simulink model "pratica2_1_b"  (R2021a)
settings: Solver=VariableStepAuto  StartTime=0.0  StopTime=10.0  RelTol=1e-3
libraries: fl_lib x11, ee_lib x7, nesl_utility x2
settings Model: Creator=ribeiro  LastModifiedBy=ribeiro

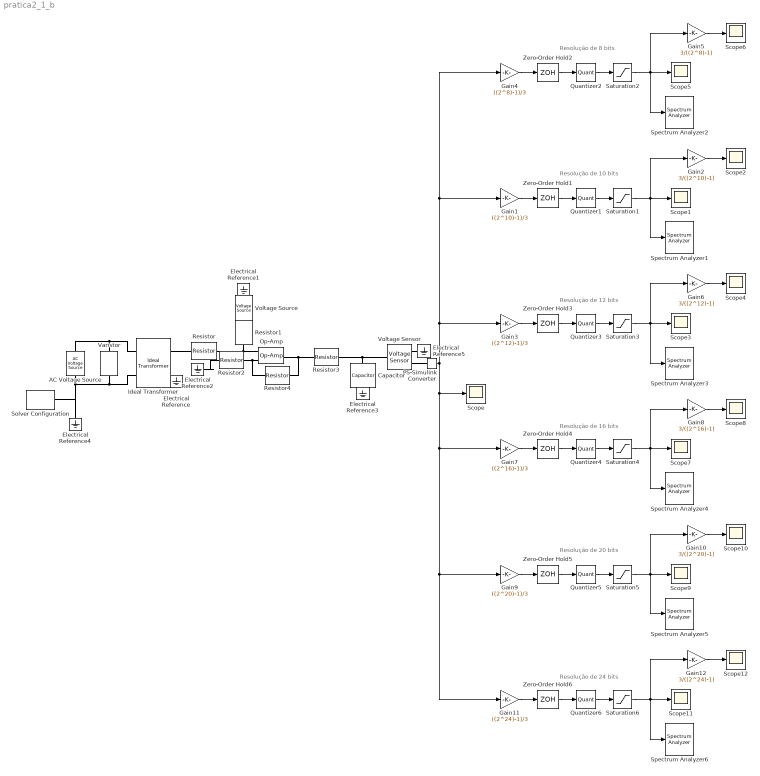
== system pratica2_1_b ==
  note: Resolução de 8 bits
  note: Resolução de 10 bits
  note: Resolução de 12 bits
  note: Resolução de 16 bits
  note: Resolução de 20 bits
  note: Resolução de 24 bits
  AC Voltage Source : fl_lib/Electrical/Electrical Sources/AC Voltage Source  amp=180 V  shift=0 deg  frequency=60 Hz  omega=0 rad/s
  Capacitor : fl_lib/Electrical/Electrical Elements/Capacitor  c=3.2 uF  r=1e-6 Ohm  g=0 1/Ohm  i_specify=off  i_priority=None  i=0 A  i_nominal_specify=off  i_nominal_unit=A  i_nominal_value=1  v_specify=off  v_priority=None  v=0 V  v_nominal_specify=off  v_nominal_unit=V  v_nominal_value=1  vc_specify=off  vc_priority=High  vc=0 V  vc_nominal_specify=off  vc_nominal_unit=V  vc_nominal_value=1
  Electrical Reference{,1..5} (6 alike) : fl_lib/Electrical/Electrical Elements/Electrical Reference
  Gain1 : Gain  Gain=((2^10)-1)/3
  Gain10 : Gain  Gain=3/((2^20)-1)
  Gain11 : Gain  Gain=((2^24)-1)/3
  Gain12 : Gain  Gain=3/((2^24)-1)
  Gain2 : Gain  Gain=3/((2^10)-1)
  Gain3 : Gain  Gain=((2^12)-1)/3
  Gain4 : Gain  Gain=((2^8)-1)/3
  Gain5 : Gain  Gain=3/((2^8)-1)
  Gain6 : Gain  Gain=3/((2^12)-1)
  Gain7 : Gain  Gain=((2^16)-1)/3
  Gain8 : Gain  Gain=3/((2^16)-1)
  Gain9 : Gain  Gain=((2^20)-1)/3
  Ideal Transformer : fl_lib/Electrical/Electrical Elements/Ideal Transformer  n=120/1  i1_specify=off  i1_priority=None  i1=0 A  i1_nominal_specify=off  i1_nominal_unit=A  i1_nominal_value=1  v1_specify=off  v1_priority=None  v1=0 V  v1_nominal_specify=off  v1_nominal_unit=V  v1_nominal_value=1  i2_specify=off  i2_priority=None  i2=0 A  i2_nominal_specify=off  i2_nominal_unit=A  i2_nominal_value=1  v2_specify=off  v2_priority=None  v2=0 V  v2_nominal_specify=off  v2_nominal_unit=V  v2_nominal_value=1
      settings: SourceProductBaseCode=SS
  Op-Amp : fl_lib/Electrical/Electrical Elements/Op-Amp  outI_specify=off  outI_priority=None  outI=0 A  outI_nominal_specify=off  outI_nominal_unit=A  outI_nominal_value=1
  PS-Simulink Converter : nesl_utility/PS-Simulink Converter  PhysicalDomain=network_engine_domain  SubClassName=ps_output  LeftPortType=input  RightPortType=output  PseudoPeriodic=off  Frequencies=[]  Unit=inherit  AffineConversion=off
      settings: SourceProductBaseCode=PW,SS
  Quantizer1 : Quantizer  QuantizationInterval=1/((2^10)-1)
  Quantizer2 : Quantizer  QuantizationInterval=1/((2^8)-1)
  Quantizer3 : Quantizer  QuantizationInterval=1/((2^12)-1)
  Quantizer4 : Quantizer  QuantizationInterval=1/((2^16)-1)
  Quantizer5 : Quantizer  QuantizationInterval=1/((2^20)-1)
  Quantizer6 : Quantizer  QuantizationInterval=1/((2^24)-1)
  Resistor : ee_lib/Passive/Resistor  R=10 kOhm  R_tol=5  enable_R_tol=0  tol_distribution=1  nSigma=4  enable_operating_limits=0  operating_limit_action=2  max_working_voltage=100 V  power_rating=1 W  enable_faults=0  fault_action=1  R_faulted=inf Ohm  enable_temporal_fault=0  t_fault=1 s  enable_behavioral_fault=0  max_permissible_current=1 A  t_fail_on_current=1 s  noise_mode=0  sample_time=1e-3 s  repeatability=1  auto_seed=3546856910  user_seed=0  Tdevice=25 degC  alpha=3.93e-3 1/K  Tmeas=25 degC  thermal_mass=100 J/K  power_derating_T1=70 degC  power_derating_T2=155 degC  operating_temperature_range_vec=[-50, 150] degC  temperature_specify=off  temperature_priority=High  temperature=298.15 K  temperature_nominal_specify=off  temperature_nominal_unit=K  temperature_nominal_value=1
  Resistor1 : ee_lib/Passive/Resistor  R=10 kOhm  R_tol=5  enable_R_tol=0  tol_distribution=1  nSigma=4  enable_operating_limits=0  operating_limit_action=2  max_working_voltage=100 V  power_rating=1 W  enable_faults=0  fault_action=1  R_faulted=inf Ohm  enable_temporal_fault=0  t_fault=1 s  enable_behavioral_fault=0  max_permissible_current=1 A  t_fail_on_current=1 s  noise_mode=0  sample_time=1e-3 s  repeatability=1  auto_seed=3198431252  user_seed=0  Tdevice=25 degC  alpha=3.93e-3 1/K  Tmeas=25 degC  thermal_mass=100 J/K  power_derating_T1=70 degC  power_derating_T2=155 degC  operating_temperature_range_vec=[-50, 150] degC  temperature_specify=off  temperature_priority=High  temperature=298.15 K  temperature_nominal_specify=off  temperature_nominal_unit=K  temperature_nominal_value=1
  Resistor2 : ee_lib/Passive/Resistor  R=10 kOhm  R_tol=5  enable_R_tol=0  tol_distribution=1  nSigma=4  enable_operating_limits=0  operating_limit_action=2  max_working_voltage=100 V  power_rating=1 W  enable_faults=0  fault_action=1  R_faulted=inf Ohm  enable_temporal_fault=0  t_fault=1 s  enable_behavioral_fault=0  max_permissible_current=1 A  t_fail_on_current=1 s  noise_mode=0  sample_time=1e-3 s  repeatability=1  auto_seed=1247433155  user_seed=0  Tdevice=25 degC  alpha=3.93e-3 1/K  Tmeas=25 degC  thermal_mass=100 J/K  power_derating_T1=70 degC  power_derating_T2=155 degC  operating_temperature_range_vec=[-50, 150] degC  temperature_specify=off  temperature_priority=High  temperature=298.15 K  temperature_nominal_specify=off  temperature_nominal_unit=K  temperature_nominal_value=1
  Resistor3 : ee_lib/Passive/Resistor  R=100 Ohm  R_tol=5  enable_R_tol=0  tol_distribution=1  nSigma=4  enable_operating_limits=0  operating_limit_action=2  max_working_voltage=100 V  power_rating=1 W  enable_faults=0  fault_action=1  R_faulted=inf Ohm  enable_temporal_fault=0  t_fault=1 s  enable_behavioral_fault=0  max_permissible_current=1 A  t_fail_on_current=1 s  noise_mode=0  sample_time=1e-3 s  repeatability=1  auto_seed=1043031083  user_seed=0  Tdevice=25 degC  alpha=3.93e-3 1/K  Tmeas=25 degC  thermal_mass=100 J/K  power_derating_T1=70 degC  power_derating_T2=155 degC  operating_temperature_range_vec=[-50, 150] degC  temperature_specify=off  temperature_priority=High  temperature=298.15 K  temperature_nominal_specify=off  temperature_nominal_unit=K  temperature_nominal_value=1
  Resistor4 : ee_lib/Passive/Resistor  R=10 kOhm  R_tol=5  enable_R_tol=0  tol_distribution=1  nSigma=4  enable_operating_limits=0  operating_limit_action=2  max_working_voltage=100 V  power_rating=1 W  enable_faults=0  fault_action=1  R_faulted=inf Ohm  enable_temporal_fault=0  t_fault=1 s  enable_behavioral_fault=0  max_permissible_current=1 A  t_fail_on_current=1 s  noise_mode=0  sample_time=1e-3 s  repeatability=1  auto_seed=3940307545  user_seed=0  Tdevice=25 degC  alpha=3.93e-3 1/K  Tmeas=25 degC  thermal_mass=100 J/K  power_derating_T1=70 degC  power_derating_T2=155 degC  operating_temperature_range_vec=[-50, 150] degC  temperature_specify=off  temperature_priority=High  temperature=298.15 K  temperature_nominal_specify=off  temperature_nominal_unit=K  temperature_nominal_value=1
  Saturation1 : Saturate  UpperLimit=(2^10)-1  LowerLimit=0
  Saturation2 : Saturate  UpperLimit=(2^8)-1  LowerLimit=0
  Saturation3 : Saturate  UpperLimit=(2^12)-1  LowerLimit=0
  Saturation4 : Saturate  UpperLimit=(2^16)-1  LowerLimit=0
  Saturation5 : Saturate  UpperLimit=(2^20)-1  LowerLimit=0
  Saturation6 : Saturate  UpperLimit=(2^24)-1  LowerLimit=0
  Scope{,1..12} (13 alike) : Scope
  Solver Configuration : nesl_utility/Solver Configuration  PhysicalDomain=network_engine_domain  SubClassName=solver  LeftPortType=input  RightPortType=generic  Tones=[]  Harmonics=[]  SimulateNoise=off  Profile=off  UseLocalSampling=off  EnableSwitchedLinearOptims=on  FrequencyDomain=off  UseCCode=off  RelTol=0.001  AbsTol=1e-06  MinStep=1e-09  ToWorkspace=off  RevertToSquareIcSolve=off  NumHomotopyIterations=100  PhasorMode=off  PhasorModeNumHarmonics=1  DoDC=off  ResidualTolerance=1e-09  UseLocalSolver=off  LocalSolverChoice=NE_BACKWARD_EULER_ADVANCER  LocalSolverSampleTime=0.001  DoFixedCost=off  MaxNonlinIter=3  MaxModeIter=2  ComputeImpulses=off  ImpulseIterations=2  LinearAlgebra=auto  EquationFormulation=NE_TIME_EF  DelaysMemoryBudget=1024  AutomaticFiltering=on  FilteringTimeConstant=0.001  PartitionStorageMethod=AS_NEEDED  PartitionMemoryBudget=1024  PartitionMethod=ROBUST
      settings: SourceProductBaseCode=PW,SS
  Spectrum Analyzer{1..6} (6 alike) : SpectrumAnalyzer
  Varistor : ee_lib/Passive/Varistor  prm=1  vclamp=260 V  roff=3e8 Ohm  ron=1 Ohm  vln=130 V  vnu=300 V  rLeak=3e8 Ohm  alphaNormal=45  rUpturn=0.07 Ohm  rseries=100e-6 Ohm  c=4.4 nF  v_varistor_specify=off  v_varistor_priority=None  v_varistor=0 V  v_varistor_nominal_specify=off  v_varistor_nominal_unit=V  v_varistor_nominal_value=1
      settings: SourceProductBaseCode=PS  InternalSimscapePortConfiguration="{\"Bottom\":[],\"Left\":[{\"id\":\"p\",\"label\":\"+\",\"type\":\"foundation.electrical.electrical\"}],\"Right\":[{\"id\":\"n\",\"label\":\"-\",\"type\":\"foundation.electrical.electrical\"}],\"Top\":[]}"
  Voltage Sensor : fl_lib/Electrical/Electrical Sensors/Voltage Sensor
  Voltage Source : ee_lib/Sources/Voltage Source  dc_voltage=1.5 V  ac_voltage=0 V  ac_shift=0 rad  ac_frequency=60 Hz  noise_mode=0  PSD=0 V^2/Hz  repeatability=1  auto_seed=3992639680  user_seed=0  sample_time=1e-3 s  i_specify=off  i_priority=None  i=0 A  i_nominal_specify=off  i_nominal_unit=A  i_nominal_value=1  v_specify=off  v_priority=None  v=0 V  v_nominal_specify=off  v_nominal_unit=V  v_nominal_value=1
  Zero-Order Hold{1..6} (6 alike) : ZeroOrderHold  SampleTime=1/1200
  wires:
  PS-Simulink Converter/1 -> Gain3/1, Gain1/1, Gain4/1, Gain11/1, Gain9/1, Gain7/1, Scope/1
  Gain5/1 -> Scope6/1
  Saturation2/1 -> Gain5/1, Spectrum Analyzer2/1, Scope5/1
  Quantizer2/1 -> Saturation2/1
  Zero-Order Hold2/1 -> Quantizer2/1
  Gain4/1 -> Zero-Order Hold2/1
  Saturation1/1 -> Gain2/1, Spectrum Analyzer1/1, Scope1/1
  Gain1/1 -> Zero-Order Hold1/1
  Zero-Order Hold1/1 -> Quantizer1/1
  Gain2/1 -> Scope2/1
  Quantizer1/1 -> Saturation1/1
  Saturation3/1 -> Gain6/1, Spectrum Analyzer3/1, Scope3/1
  Gain3/1 -> Zero-Order Hold3/1
  Zero-Order Hold3/1 -> Quantizer3/1
  Gain6/1 -> Scope4/1
  Quantizer3/1 -> Saturation3/1
  Saturation4/1 -> Gain8/1, Spectrum Analyzer4/1, Scope7/1
  Gain7/1 -> Zero-Order Hold4/1
  Zero-Order Hold4/1 -> Quantizer4/1
  Gain8/1 -> Scope8/1
  Quantizer4/1 -> Saturation4/1
  Saturation5/1 -> Gain10/1, Spectrum Analyzer5/1, Scope9/1
  Gain9/1 -> Zero-Order Hold5/1
  Zero-Order Hold5/1 -> Quantizer5/1
  Gain10/1 -> Scope10/1
  Quantizer5/1 -> Saturation5/1
  Saturation6/1 -> Gain12/1, Spectrum Analyzer6/1, Scope11/1
  Gain11/1 -> Zero-Order Hold6/1
  Zero-Order Hold6/1 -> Quantizer6/1
  Gain12/1 -> Scope12/1
  Quantizer6/1 -> Saturation6/1
  connections:
  AC Voltage Source/LConn1 -- Ideal Transformer/LConn1 -- Varistor/LConn1
  AC Voltage Source/RConn1 -- Solver Configuration/RConn1 -- Electrical Reference4/LConn1 -- Ideal Transformer/LConn2 -- Varistor/RConn1
  Resistor/LConn1 -- Ideal Transformer/RConn1
  Ideal Transformer/RConn2 -- Electrical Reference/LConn1
  Electrical Reference2/LConn1 -- Resistor2/LConn1
  Op-Amp/LConn1 -- Resistor1/LConn1 -- Resistor/RConn1
  Op-Amp/RConn1 -- Resistor4/RConn1 -- Resistor3/LConn1
  Resistor2/RConn1 -- Resistor4/LConn1 -- Op-Amp/LConn2
  Resistor3/RConn1 -- Voltage Sensor/LConn1 -- Capacitor/LConn1
  Electrical Reference3/LConn1 -- Capacitor/RConn1
  Electrical Reference5/LConn1 -- Voltage Sensor/RConn2
  Voltage Sensor/RConn1 -- PS-Simulink Converter/LConn1
  Voltage Source/LConn1 -- Resistor1/RConn1
  Electrical Reference1/LConn1 -- Voltage Source/RConn1
